simulink model "RectifierBuckConverterTopology_Shunt"  (R2021b)
settings: Solver=VariableStepAuto  StartTime=0.0  StopTime=3  MaxStep=1e-6  RelTol=1e-3
libraries: spsDiodeLib x7, spsACVoltageSourceLib x3, spsMeanLib x2, spsVoltageMeasurementLib x2, spsCurrentMeasurementLib x1, spsDCMachineLib x1, spsGroundLib x1, spsMosfetLib x1, eePowerMeasurement x1, spsSeriesRLCBranchLib x1, spspowerguiLib x1
settings Model: Creator=pc3  LastModifiedBy=Burnie Barren
settings SolverCC: ZeroCrossAlgorithm=Adaptive
settings DebuggingCC: IgnoredZcDiagnostic=none

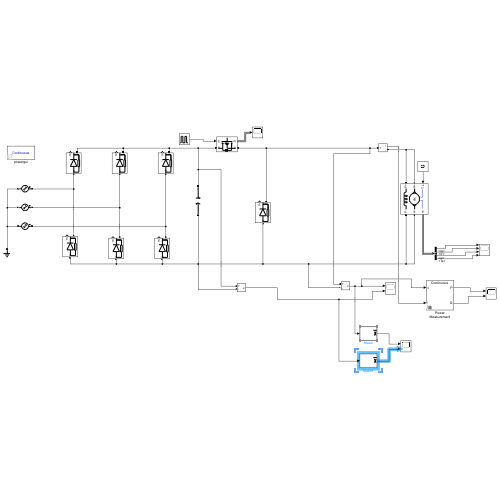
[thumbnail: Simulink's stored preview of the top-level diagram]
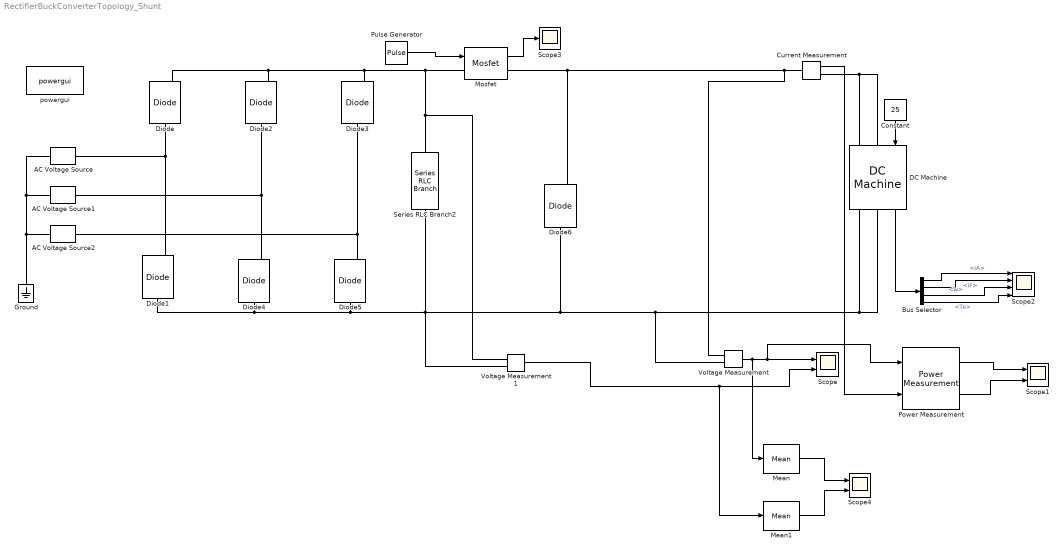
== system RectifierBuckConverterTopology_Shunt ==
  AC Voltage Source : spsACVoltageSourceLib/AC Voltage Source  Amplitude=125*sqrt(2)  Phase=0  Frequency=50  SampleTime=0  Measurements=None  BusType=swing  Pref=10e3  Qref=0  Qmin=-inf  Qmax=+inf
  AC Voltage Source1 : spsACVoltageSourceLib/AC Voltage Source  Amplitude=125*sqrt(2)  Phase=120  Frequency=50  SampleTime=0  Measurements=None  BusType=swing  Pref=10e3  Qref=0  Qmin=-inf  Qmax=+inf
  AC Voltage Source2 : spsACVoltageSourceLib/AC Voltage Source  Amplitude=125*sqrt(2)  Phase=240  Frequency=50  SampleTime=0  Measurements=None  BusType=swing  Pref=10e3  Qref=0  Qmin=-inf  Qmax=+inf
  Bus Selector : BusSelector  OutputSignals=iA,iF,w,Te
  Constant : Constant  Value=25
  Current Measurement : spsCurrentMeasurementLib/Current Measurement  PhasorSimulation=off  OutputType=Complex  PSBequivalent=0
  DC Machine : spsDCMachineLib/DC Machine  PresetModel=No  MechanicalLoad=Torque TL  FieldType=Wound  ShowDetailedParameters=on  MeasurementBus=on  RLa="[ 0.8  0.0125]"  RLf="[ 210  23]"  Laf=1.8  MachineConstant=Torque constant (N.m/A)  Ke=1.8  Kt=1.8  J=1  Bm=0  Tf=0  w0=0  Ifinit=1.18334920786918e-19  TsPowergui=0  TsBlock=-1
  Diode{,1..5} (6 alike) : spsDiodeLib/Diode  Ron=0.001  Lon=0  Vf=1.2  IC=0  UseSnubber=0  Rs=500  Cs=250e-9  Measurements=on
  Diode6 : spsDiodeLib/Diode  Ron=0.001  Lon=0  Vf=0.8  IC=0  UseSnubber=0  Rs=500  Cs=250e-9  Measurements=on
  Ground : spsGroundLib/Ground  LConnTagsString=a
  Mean : spsMeanLib/Mean  Freq=50  Vinit=0  Ts=0
  Mean1 : spsMeanLib/Mean  Freq=50  Vinit=0  Ts=0
  Mosfet : spsMosfetLib/Mosfet  Ron=0.1  Lon=0  Rd=0.01  Vfd=0  IC=0  Rs=1e5  Cs=inf  Measurements=on
  Power Measurement : eePowerMeasurement/Power Measurement  LabelModeActiveChoice=Continuous  F=50  K=[0 1 2 3]  Ts=0
      settings: SourceProductBaseCode=PS
  Pulse Generator : DiscretePulseGenerator  PulseType=Time based  Amplitude=12  Period=0.1e-3  PulseWidth=50
  Scope : Scope  NumInputPorts=2
  Scope1 : Scope  NumInputPorts=2
  Scope2 : Scope  NumInputPorts=4
  Scope3 : Scope
  Scope4 : Scope  NumInputPorts=2
  Series RLC Branch2 : spsSeriesRLCBranchLib/Series RLC Branch  LConnTagsString=__new0  RConnTagsString=__new0  BranchType=C  Resistance=1  Inductance=1e-3  SetiL0=off  InitialCurrent=0  Capacitance=1e-3  Setx0=off  InitialVoltage=0  Measurements=None
  Voltage Measurement : spsVoltageMeasurementLib/Voltage Measurement  PhasorSimulation=off  OutputType=Complex  PSBequivalent=0
  Voltage Measurement1 : spsVoltageMeasurementLib/Voltage Measurement  PhasorSimulation=off  OutputType=Complex  PSBequivalent=0
  powergui : spspowerguiLib/powergui  Priority=1  SimulationMode=Continuous  SampleTime=50e-6  frequency=60  Iterations=50  frequencyindice=50  Pbase=100e6  ErrMax=1e-4  UnitsV=kV  UnitsW=MW  buscounter=0  FunctionMessages=off  echomessages=off  EnableUseOfTLC=off  CurrentSourceSwitches=off  DisableSnubberDevices=off  DisableRonSwitches=off  DisableVfSwitches=off  DisplayEquations=off  AutomaticDiscreteSolvers=off  SolverType=Tustin/Backward Euler (TBE)  Interpol=off  ExternalGateDelay=off  methode=off  Ts=100  x0status=blocks  SPID=on  SwTol=0  HookPort=off  NonlinearTolerance=1e-4  nMaxIteration=100  ContinueOnMaxIteration=off  RestoreLinks=warning  ResistiveCurrentMeasurement=off  Frange=[0:2:500]  Ylog=off  Xlog=on  ShowGrid=off  save=off  variable=ZData  structure=0  ZoomFFT=off  StartTime=0.0  cycles=1  DisplayStyle=1  fundamental=60  FreqAxis=off  MaxFrequency=1000  frequencyindicesteady=1  RmsSteady=1  display=off
  wires:
  Pulse Generator/1 -> Mosfet/1
  Constant/1 -> DC Machine/1
  DC Machine/1 -> Bus Selector/1
  Voltage Measurement/1 -> Mean/1, Scope/1, Power Measurement/1
  Current Measurement/1 -> Power Measurement/2
  Power Measurement/1 -> Scope1/1
  Power Measurement/2 -> Scope1/2
  Voltage Measurement1/1 -> Mean1/1, Scope/2
  Bus Selector/1 -> Scope2/1  "<iA>"
  Bus Selector/2 -> Scope2/2  "<iF>"
  Bus Selector/3 -> Scope2/3  "<w>"
  Bus Selector/4 -> Scope2/4  "<Te>"
  Mosfet/1 -> Scope3/1
  Mean/1 -> Scope4/1
  Mean1/1 -> Scope4/2
  connections:
  Ground/LConn1 -- AC Voltage Source2/LConn1 -- AC Voltage Source1/LConn1 -- AC Voltage Source/LConn1
  Diode5/RConn1 -- AC Voltage Source2/RConn1 -- Diode3/LConn1
  Diode4/RConn1 -- AC Voltage Source1/RConn1 -- Diode2/LConn1
  Diode/LConn1 -- Diode1/RConn1 -- AC Voltage Source/RConn1
  Diode/RConn1 -- Voltage Measurement1/LConn1 -- Series RLC Branch2/LConn1 -- Mosfet/LConn1 -- Diode3/RConn1 -- Diode2/RConn1
  Diode6/RConn1 -- Current Measurement/LConn1 -- Voltage Measurement/LConn1 -- Mosfet/RConn1
  DC Machine/LConn1 -- Current Measurement/RConn1 -- DC Machine/LConn2
  Voltage Measurement/LConn2 -- DC Machine/RConn1 -- DC Machine/RConn2 -- Series RLC Branch2/RConn1 -- Voltage Measurement1/LConn2 -- Diode1/LConn1 -- Diode4/LConn1 -- Diode5/LConn1 -- Diode6/LConn1
